simulink model "buck_12v_to_5v_100khz"  (R2024b)
settings: Solver=ode23t  StartTime=0.0  StopTime=0.004  MaxStep=1e-7  RelTol=1e-3
model workspace (MAT data in the model file):
  buck_C = 0.0001
  buck_L = 0.0001
  buck_duty = 0.416666666667
  buck_fsw = 100000
  buck_loadR = 10
  buck_vin = 12
  buck_vout_target = 5
libraries: fl_lib x7, nesl_utility x3, ee_lib x1
settings Model: Creator=yang  LastModifiedBy=yang

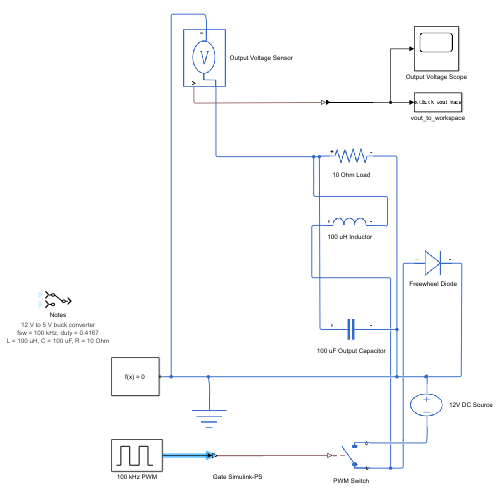
[thumbnail: Simulink's stored preview of the top-level diagram]
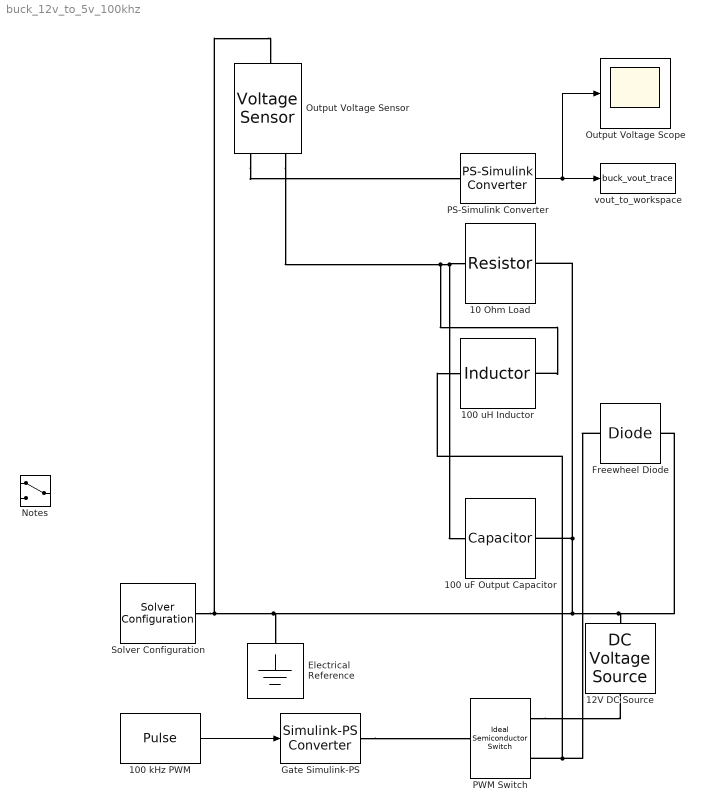
== system buck_12v_to_5v_100khz ==
  10 Ohm Load : fl_lib/Electrical/Electrical Elements/Resistor  R=10 Ohm  i_specify=off  i_priority=None  i=0 A  i_nominal_specify=off  i_nominal_value=1  i_nominal_unit=A  v_specify=off  v_priority=None  v=0 V  v_nominal_specify=off  v_nominal_value=1  v_nominal_unit=V
  100 kHz PWM : DiscretePulseGenerator  PulseType=Time based  Period=1e-05  PulseWidth=41.6666666666667  SampleTime=0
  100 uF Output Capacitor : fl_lib/Electrical/Electrical Elements/Capacitor  c=0.0001 F  r=0.02 Ohm  g=1e-9 1/Ohm  i_specify=off  i_priority=None  i=0 A  i_nominal_specify=off  i_nominal_value=1  i_nominal_unit=A  v_specify=off  v_priority=None  v=0 V  v_nominal_specify=off  v_nominal_value=1  v_nominal_unit=V  vc_specify=off  vc_priority=High  vc=0 V  vc_nominal_specify=off  vc_nominal_value=1  vc_nominal_unit=V
  100 uH Inductor : fl_lib/Electrical/Electrical Elements/Inductor  l=0.0001 H  r=0.02 Ohm  g=1e-9 1/Ohm  i_specify=off  i_priority=None  i=0 A  i_nominal_specify=off  i_nominal_value=1  i_nominal_unit=A  v_specify=off  v_priority=None  v=0 V  v_nominal_specify=off  v_nominal_value=1  v_nominal_unit=V  i_L_specify=off  i_L_priority=High  i_L=0 A  i_L_nominal_specify=off  i_L_nominal_value=1  i_L_nominal_unit=A
  12V DC Source : fl_lib/Electrical/Electrical Sources/DC Voltage Source  v0=12 V
  Electrical Reference : fl_lib/Electrical/Electrical Elements/Electrical Reference
  Freewheel Diode : fl_lib/Electrical/Electrical Elements/Diode  Vf=0.4 V  Ron=1e-3 Ohm  Goff=1e-6 1/Ohm  i_specify=off  i_priority=None  i=0 A  i_nominal_specify=off  i_nominal_value=1  i_nominal_unit=A  v_specify=off  v_priority=None  v=0 V  v_nominal_specify=off  v_nominal_value=1  v_nominal_unit=V
  Gate Simulink-PS : nesl_utility/Simulink-PS Converter  PhysicalDomain=network_engine_domain  SubClassName=ps_input  LeftPortType=input  RightPortType=output  PseudoPeriodic=off  Frequencies=[]  NoiseDistribution=none  NoiseParameters=[]  Unit=V  AffineConversion=off  FilteringAndDerivatives=provide  SimscapeFilterOrder=1  InputFilterTimeConstant=0.001  UdotUserProvided=0
  Notes : ManualSwitch
      settings: AttributesFormatString=12 V to 5 V buck converter\nfsw = 100 kHz, duty = 0.4167\nL = 100 uH, C = 100 uF, R = 10 Ohm
  Output Voltage Scope : Scope
  Output Voltage Sensor : fl_lib/Electrical/Electrical Sensors/Voltage Sensor
  PS-Simulink Converter : nesl_utility/PS-Simulink Converter  PhysicalDomain=network_engine_domain  SubClassName=ps_output  LeftPortType=input  RightPortType=output  PseudoPeriodic=off  Frequencies=[]  VectorFormat=inherit  Unit=V  AffineConversion=off
  PWM Switch : ee_lib/Semiconductors & Converters/Ideal Semiconductor Switch  port_option=ee.enum.controlport.ps  Ron=1e-3 Ohm  Goff=1e-6 1/Ohm  Vth=0.5 V  diode_param=ee.enum.semiconductors.protectionDiode.external  diode_Vf=0.8 V  diode_Ron=0.001 Ohm  diode_Goff=1e-5 1/Ohm  diode_C=50e-9 F  diode_iRM=-235 A  diode_iF=300 A  diode_idot=-50 A/us  diode_trr_param=ee.enum.converters.diodetrr.trr_factor  diode_trr_factor=3  diode_trr=15 us  diode_Qrr=1500 s*uA
  Solver Configuration : nesl_utility/Solver Configuration  PhysicalDomain=network_engine_domain  SubClassName=solver  LeftPortType=input  RightPortType=generic  Tones=[]  Harmonics=[]  SimulateNoise=off  Profile=off  UseLocalSampling=off  EnableSwitchedLinearOptims=on  FrequencyDomain=off  UseCCode=off  RelTol=0.001  AbsTol=0.001  MinStep=1e-09  ToWorkspace=off  RevertToSquareIcSolve=off  NumHomotopyIterations=100  PhasorMode=off  PhasorModeNumHarmonics=1  ConsistencySolver=NEWTON_XTOL_AFTER_FTOL  IndexReductionMethod=DerivativeReplacement  DoDC=off  ResidualTolerance=1e-09  ConsistencyTolSource=GLOBAL  ConsistencyAbsTol=0.001  ConsistencyRelTol=0.001  ConsistencyTolFactor=0.001  UseLocalSolver=off  LocalSolverChoice=NE_BACKWARD_EULER_ADVANCER  ResolveIndetEquations=on  FunctionEvalNumThread=1  LocalSolverSampleTime=0.001  DoFixedCost=off  MaxNonlinIter=3  MaxModeIter=2  ComputeImpulses=off  ImpulseIterations=2  LinearAlgebra=auto  LinearAlgebraNumThread=0  EquationFormulation=NE_TIME_EF  DelaysMemoryBudget=1024  AutomaticFiltering=on  FilteringTimeConstant=0.001  PartitionStorageMethod=AS_NEEDED  PartitionMemoryBudget=1024  PartitionMethod=ROBUST  MultibodyUseLocalSolver=off  MultibodyLocalSolverChoice=ODE1  MultibodyLocalSolverSampleTime=0.001
  vout_to_workspace : ToWorkspace  VariableName=buck_vout_trace  SaveFormat=Timeseries  SampleTime=-1
  wires:
  100 kHz PWM/1 -> Gate Simulink-PS/1
  PS-Simulink Converter/1 -> Output Voltage Scope/1, vout_to_workspace/1
  connections:
  Gate Simulink-PS/RConn1 -- PWM Switch/LConn1
  Solver Configuration/RConn1 -- Freewheel Diode/RConn1 -- 12V DC Source/LConn1 -- 100 uF Output Capacitor/RConn1 -- 10 Ohm Load/RConn1 -- Electrical Reference/LConn1 -- Output Voltage Sensor/LConn1
  Output Voltage Sensor/RConn2 -- 100 uF Output Capacitor/LConn1 -- 10 Ohm Load/LConn1 -- 100 uH Inductor/RConn1
  PWM Switch/RConn1 -- 12V DC Source/RConn1
  Output Voltage Sensor/RConn1 -- PS-Simulink Converter/LConn1
  Freewheel Diode/LConn1 -- PWM Switch/RConn2 -- 100 uH Inductor/LConn1
